simulink model "Full_Wave_Rectifier_DC_Motor"  (R2024b)
settings: Solver=ode23tb  StartTime=0.0  StopTime=2  FixedStep=1e-6  MaxStep=1e-6  RelTol=1e-3
values from neighbouring files (symbols this model uses):
  A = [-R/L -Kb/L 0; Kt/J -B/J 0; 0 1 0]    [Parameters.m]
libraries: spsThyristorLib x4, spsVoltageMeasurementLib x3, spsACVoltageSourceLib x1, spsDiodeLib x1, spsGroundLib x1, spsSeriesRLCBranchLib x1, spsDCMachineLib x1, spsDCVoltageSourceLib x1, spspowerguiLib x1
settings Model: Creator=Nabil  LastModifiedBy=Nabil

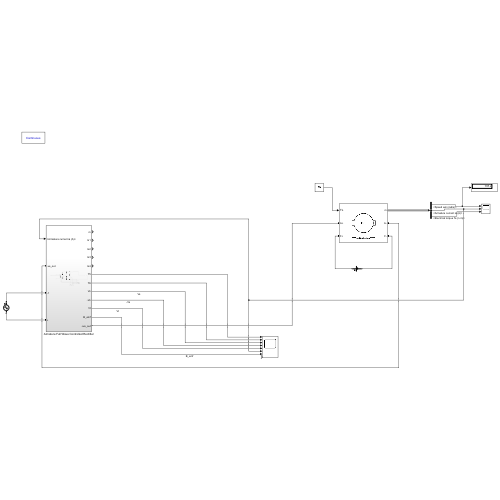
[thumbnail: Simulink's stored preview of the top-level diagram]
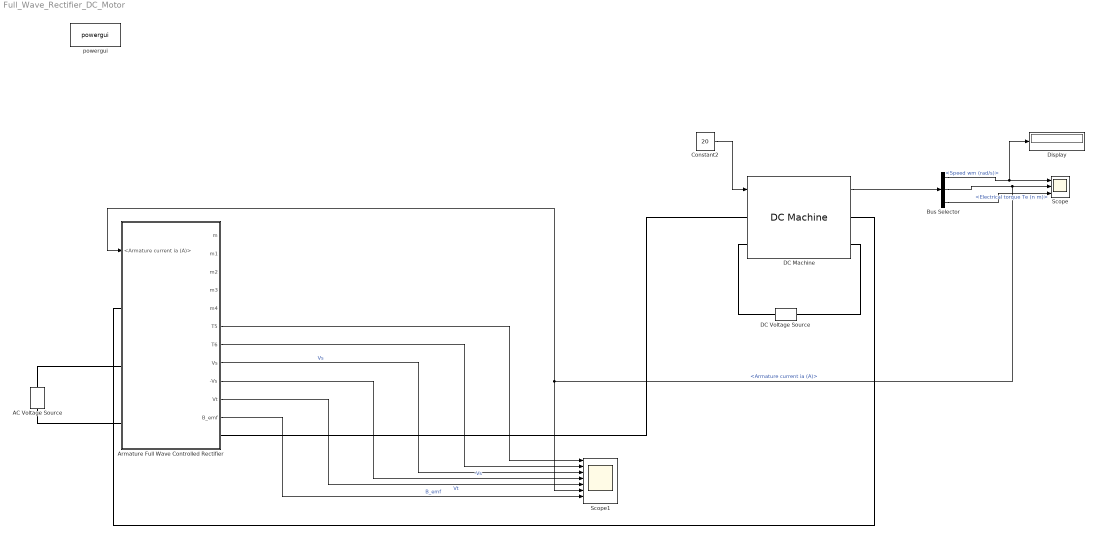
== system Full_Wave_Rectifier_DC_Motor ==
  AC Voltage Source : spsACVoltageSourceLib/AC Voltage Source  Amplitude=200  Phase=0  Frequency=50  SampleTime=0  Measurements=None  BusType=swing  Pref=10e3  Qref=0  Qmin=-inf  Qmax=+inf
  Armature Full Wave Controlled Rectifier : Subsystem
  Bus Selector : BusSelector  OutputSignals=Speed wm (rad/s),Armature current ia (A),Electrical torque Te (n m)
  Constant2 : Constant  Value=20
  DC Machine : spsDCMachineLib/DC Machine  PresetModel=04: 10HP 240V 1750RPM Field:300V  MechanicalLoad=Torque TL  FieldType=Wound  ShowDetailedParameters=on  MeasurementBus=off  RLa=[1.086 0.01216]  RLf=[180 71.47]  Laf=0.6458  MachineConstant=Torque constant (N.m/A)  Ke=1.8  Kt=1.8  J=0.04251  Bm=0.003406  Tf=1.046  w0=1  Ifinit=-5.46413480420564e-18  TsPowergui=0  TsBlock=-1
  DC Voltage Source : spsDCVoltageSourceLib/DC Voltage Source  Amplitude=300  Measurements=None
  Display : Display
  Scope : Scope  NumInputPorts=3
  Scope1 : Scope  NumInputPorts=8
  powergui : spspowerguiLib/powergui  Priority=1  SimulationMode=Continuous  SampleTime=50e-6  frequency=60  Iterations=50  frequencyindice=50  Pbase=100e6  ErrMax=1e-4  UnitsV=kV  UnitsW=MW  buscounter=0  FunctionMessages=off  echomessages=off  EnableUseOfTLC=off  CurrentSourceSwitches=off  DisableSnubberDevices=off  DisableRonSwitches=off  DisableVfSwitches=off  DisplayEquations=off  AutomaticDiscreteSolvers=off  SolverType=Tustin/Backward Euler (TBE)  Interpol=off  ExternalGateDelay=off  methode=off  Ts=100  x0status=blocks  SPID=on  SwTol=0  HookPort=off  NonlinearTolerance=1e-4  nMaxIteration=100  ContinueOnMaxIteration=off  RestoreLinks=warning  ResistiveCurrentMeasurement=off  Frange=[0:2:500]  Ylog=off  Xlog=on  ShowGrid=off  save=off  variable=ZData  structure=0  ZoomFFT=off  StartTime=0.0  cycles=1  DisplayStyle=1  fundamental=60  FreqAxis=off  MaxFrequency=1000  frequencyindicesteady=1  RmsSteady=1  display=off
  wires:
  Constant2/1 -> DC Machine/1
  Bus Selector/3 -> Scope/3  "<Electrical torque Te (n m)>"
  DC Machine/1 -> Bus Selector/1
  Bus Selector/1 -> Display/1, Scope/1  "<Speed wm (rad/s)>"
  Bus Selector/2 -> Armature Full Wave Controlled Rectifier/1(<Armature current ia (A)>), Scope1/6, Scope/2  "<Armature current ia (A)>"
  Armature Full Wave Controlled Rectifier/6(T5) -> Scope1/1
  Armature Full Wave Controlled Rectifier/7(T6) -> Scope1/2
  Armature Full Wave Controlled Rectifier/8(Vs) -> Scope1/3  "Vs"
  Armature Full Wave Controlled Rectifier/9(-Vs) -> Scope1/4  "-Vs"
  Armature Full Wave Controlled Rectifier/10(Vt) -> Scope1/5  "Vt"
  Armature Full Wave Controlled Rectifier/11(B_emf) -> Scope1/7  "B_emf"
  connections:
  DC Machine/LConn1 -- Armature Full Wave Controlled Rectifier/RConn1
  DC Machine/RConn1 -- Armature Full Wave Controlled Rectifier/LConn1
  AC Voltage Source/RConn1 -- Armature Full Wave Controlled Rectifier/LConn2
  AC Voltage Source/LConn1 -- Armature Full Wave Controlled Rectifier/LConn3
  DC Voltage Source/LConn1 -- DC Machine/RConn2
  DC Voltage Source/RConn1 -- DC Machine/LConn2

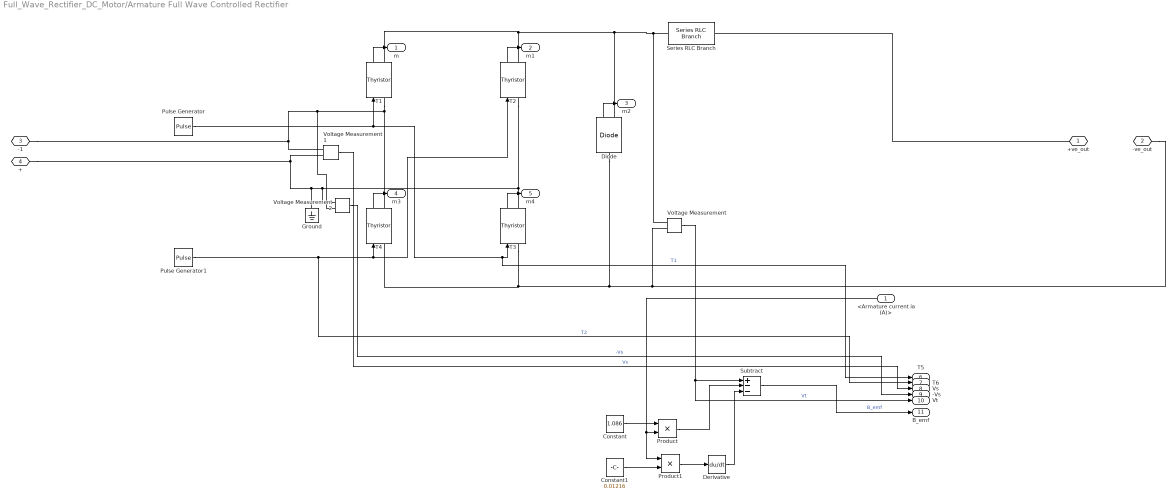
== system Full_Wave_Rectifier_DC_Motor/Armature Full Wave Controlled Rectifier ==
  <Armature current ia (A)> : Inport
  Constant : Constant  Value=1.086
  Constant1 : Constant  Value=0.01216
  Derivative : Derivative
  Diode : spsDiodeLib/Diode  Ron=0.001  Lon=0  Vf=0.8  IC=0  UseSnubber=0  Rs=500  Cs=250e-9  Measurements=on
  Ground : spsGroundLib/Ground  LConnTagsString=a
  Product : Product
  Product1 : Product
  Pulse Generator : DiscretePulseGenerator  PulseType=Time based  Period=0.02  PulseWidth=2  PhaseDelay=1.667e-3
  Pulse Generator1 : DiscretePulseGenerator  PulseType=Time based  Period=0.02  PulseWidth=2  PhaseDelay=((1.667e-3)+pi)/(100*pi)+(1.667e-3)
  Series RLC Branch : spsSeriesRLCBranchLib/Series RLC Branch  LConnTagsString=__new0  RConnTagsString=__new0  BranchType=L  Resistance=1  Inductance=5e-2  SetiL0=off  InitialCurrent=0  Capacitance=1e-6  Setx0=off  InitialVoltage=0  Measurements=None
  Subtract : Sum  Inputs=+--
  T{1..4} (4 alike) : spsThyristorLib/Thyristor  Ron=0.001  Lon=0  Vf=0.8  IC=0  Rs=500  Cs=250e-9  Measurements=on
  Voltage Measurement : spsVoltageMeasurementLib/Voltage Measurement  PhasorSimulation=off  OutputType=Complex  PSBequivalent=0
  Voltage Measurement1 : spsVoltageMeasurementLib/Voltage Measurement  PhasorSimulation=off  OutputType=Complex  PSBequivalent=0
  Voltage Measurement2 : spsVoltageMeasurementLib/Voltage Measurement  PhasorSimulation=off  OutputType=Complex  PSBequivalent=0
  +ve_out : PMIOPort  Side=Right
  -ve_out : PMIOPort  Port=2  Side=Left
  -1 : PMIOPort  Port=3  Side=Left
  + : PMIOPort  Port=4  Side=Left
  m : Outport
  m1 : Outport  Port=2
  m2 : Outport  Port=3
  m3 : Outport  Port=4
  m4 : Outport  Port=5
  T5 : Outport  Port=6
  T6 : Outport  Port=7
  Vs : Outport  Port=8
  -Vs : Outport  Port=9
  Vt : Outport  Port=10
  B_emf : Outport  Port=11
  wires:
  Constant1/1 -> Product1/2
  Pulse Generator/1 -> T1/1, T5/1, T3/1  "T1"
  T1/1 -> m/1
  T3/1 -> m4/1
  Constant/1 -> Product/1
  T2/1 -> m1/1
  Pulse Generator1/1 -> T6/1, T2/1, T4/1  "T2"
  Voltage Measurement/1 -> Vt/1, Subtract/1  "Vt"
  <Armature current ia (A)>/1 -> Product/2, Product1/1
  Voltage Measurement1/1 -> Vs/1  "Vs"
  Voltage Measurement2/1 -> -Vs/1  "-Vs"
  Diode/1 -> m2/1
  T4/1 -> m3/1
  Product1/1 -> Derivative/1
  Derivative/1 -> Subtract/3
  Product/1 -> Subtract/2
  Subtract/1 -> B_emf/1  "B_emf"
  connections:
  T1/LConn1 -- -1/RConn1 -- Voltage Measurement1/LConn1 -- Voltage Measurement2/LConn2 -- T4/RConn1
  T3/LConn1 -- -ve_out/RConn1 -- Voltage Measurement/LConn2 -- Diode/LConn1 -- T4/LConn1
  T2/LConn1 -- Voltage Measurement2/LConn1 -- +/RConn1 -- Voltage Measurement1/LConn2 -- Ground/LConn1 -- T3/RConn1
  T1/RConn1 -- Series RLC Branch/LConn1 -- Voltage Measurement/LConn1 -- Diode/RConn1 -- T2/RConn1
  +ve_out/RConn1 -- Series RLC Branch/RConn1
